simulink model "hRoseModel"  (R2015a)
settings: Solver=ode15s  StartTime=0.0  StopTime=2  RelTol=1e-3
values from neighbouring files (symbols this model uses):
  epsilon = 0.01    [hRose.m]
  fast_plant_X0 = -1.0    (= -1)    [averagedRelayOutput.m]    (also in bursting_linearised.m = -1.05; fastSlow.m; fast_nullcline_winged_cusp.m; hRose.m = 0)
  slow_plant_X0 = -1.0    (= -1)    [averagedRelayOutput.m]    (also in bursting_linearised.m = -1.05; fastSlow.m; fast_nullcline_winged_cusp.m = -2; hRose.m = -10)
  ultra_slow_plant_X0 = 0.45    [averagedRelayOutput.m]    (also in bursting_linearised.m = 0; fastSlow.m; hRose.m = 2000; manParamsNullclines.m)
settings Model: Creator=ra428  LastModifiedBy=rajiv

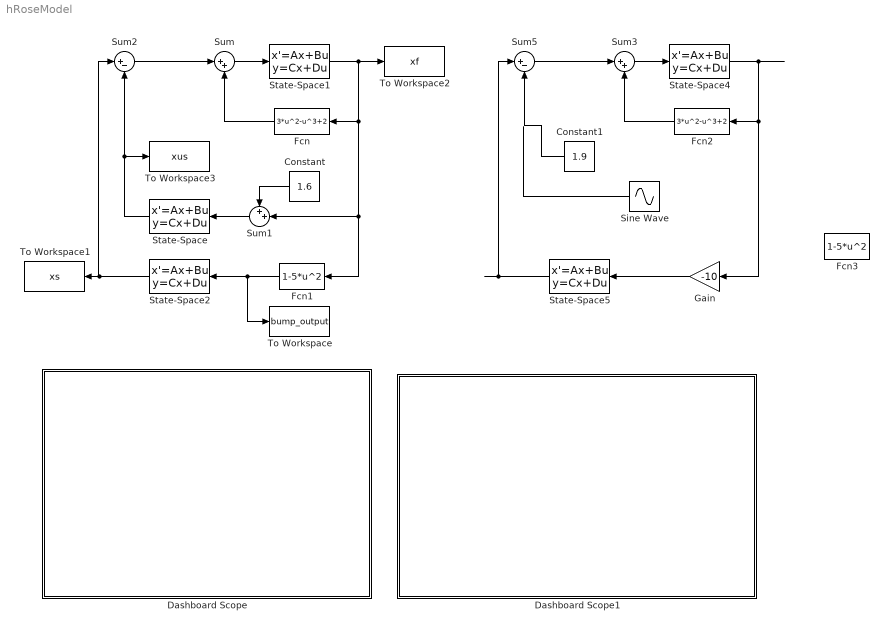
== system hRoseModel ==
  Constant : Constant  Value=1.6
  Constant1 : Constant  Value=1.9
  Dashboard Scope : Subsystem  DialogController=hmiCreateDDGDialog  IsWebBlock=on  mask(MathWorksWebBlock){webBlockId=9e290eaa-feac-417c-9444-f83b371a34f5, webBlockType=sdiscope, ShowInitialText=on, HMISrcModelName=hRoseModel}
      mask prompts: webBlockId "WebBlock Id"; webBlockType "WebBlock Type"; HMISrcModelName "Source Model"
      mask Help: helpview([docroot '/mapfiles/simulink.map'], 'hmi_scope')
      mask Display:
      | if strcmp(get_param(bdroot(gcb),'BlockDiagramType'), 'library')
      |     image([(matlabroot) '/toolbox/simulink/hmi/icons/DashboardScope.png']);
      | end
  Dashboard Scope1 : Subsystem  DialogController=hmiCreateDDGDialog  IsWebBlock=on  mask(MWDashboardBlock){webBlockId=9f8f0b92-cc9e-437b-932f-8b750270ba14, webBlockType=sdiscope, ShowInitialText=on, HMISrcModelName=hRoseModel}
      mask prompts: webBlockId "WebBlock Id"; webBlockType "WebBlock Type"; HMISrcModelName "Source Model"
      mask Help: helpview([docroot '/mapfiles/simulink.map'], 'hmi_scope')
      mask Display:
      | if strcmp(get_param(bdroot(gcb),'BlockDiagramType'), 'library')
      |     image([(matlabroot) '/toolbox/simulink/hmi/icons/DashboardScope.png']);
      | end
  Fcn : Fcn  Expr=3*u^2-u^3+2
  Fcn1 : Fcn  Expr=1-5*u^2
  Fcn2 : Fcn  Expr=3*u^2-u^3+2
  Fcn3 : Fcn  Expr=1-5*u^2
  Gain : Gain  Gain=-10
  Sine Wave : Sin  Amplitude=0.2  Bias=1.7  SampleTime=0
  State-Space : StateSpace  A=-.001  B=4  C=0.001  D=0  X0=ultra_slow_plant_X0
  State-Space1 : StateSpace  A=0  C=1/epsilon  D=0  X0=fast_plant_X0
  State-Space2 : StateSpace  A=-1  D=0  X0=slow_plant_X0
  State-Space4 : StateSpace  A=0  C=1/epsilon  D=0  X0=0
  State-Space5 : StateSpace  A=-1  D=0  X0=0
  Sum : Sum  Inputs=|++
  Sum1 : Sum  Inputs=++|
  Sum2 : Sum  Inputs=|+-
  Sum3 : Sum  Inputs=|++
  Sum5 : Sum  Inputs=|+-
  To Workspace : ToWorkspace  VariableName=bump_output  SaveFormat=Timeseries  SampleTime=-1
  To Workspace1 : ToWorkspace  VariableName=xs  SaveFormat=Timeseries  SampleTime=-1
  To Workspace2 : ToWorkspace  VariableName=xf  SaveFormat=Timeseries  SampleTime=-1
  To Workspace3 : ToWorkspace  VariableName=xus  SaveFormat=Timeseries  SampleTime=-1
  wires:
  Sum/1 -> State-Space1/1
  Fcn/1 -> Sum/2
  State-Space1/1 -> Fcn/1, Fcn1/1, Sum1/2, To Workspace2/1
  Sum1/1 -> State-Space/1
  State-Space/1 -> To Workspace3/1, Sum2/2
  Sum2/1 -> Sum/1
  Constant/1 -> Sum1/1
  Fcn1/1 -> To Workspace/1, State-Space2/1
  State-Space2/1 -> Sum2/1, To Workspace1/1
  Sum3/1 -> State-Space4/1
  Fcn2/1 -> Sum3/2
  State-Space4/1 -> Gain/1, Fcn2/1
  Sum5/1 -> Sum3/1
  State-Space5/1 -> Sum5/1
  Sine Wave/1 -> ?
  Constant1/1 -> Sum5/2
  Gain/1 -> State-Space5/1

== system hRoseModel/Dashboard Scope ==

== system hRoseModel/Dashboard Scope1 ==
